simulink model "mc_power_model"  (R2022b)
settings: Solver=VariableStepAuto  StartTime=0.0  StopTime=5  FixedStep=1e-8  MaxStep=1e-7  RelTol=1e-3
undefined symbols (not defined in the file): f_s, find_system, Jm, Ki_ibat, Ki_id, Ki_iq, Kp_ibat, Kp_id, Kp_iq, Ld, limit_duty, Lq, p, Phi, Rs, Shunt, Snubber, Ts, U_dc, Vs_max
libraries: spsSeriesRLCBranchLib x12, spsCurrentMeasurementLib x9, spsVoltageMeasurementLib x7, spsMosfetLib x6, simulink x3, spsTriangleGeneratorLib x2, spsMeanLib x2, spsGroundLib x1, spsPermanentMagnetSynchronousMachineLib x1, spsDCVoltageSourceLib x1, spsThreePhaseVIMeasurementLib x1, spspowerguiLib x1
settings Model: Creator=ngoqu  LastModifiedBy=DoCongHieu
settings SolverCC: AlgebraicLoopSolver=TrustRegion
settings DataIOCC: ReturnWorkspaceOutputs=off
settings DebuggingCC: UnconnectedInputMsg=warning  UnconnectedOutputMsg=warning  UnconnectedLineMsg=warning  SFMachineParentedDataDiag=warning  ArithmeticOperatorsInVariantConditions=warning
settings ModelReferenceCC: EnableRefExpFcnMdlSchedulingChecks=on
settings SFSimCC: SimUseLocalCustomCode=off  CustomCodeUndefinedFunction=UseInterfaceOnly
settings RTWCC: RTWUseLocalCustomCode=off  DLArmComputeVersion=19.05

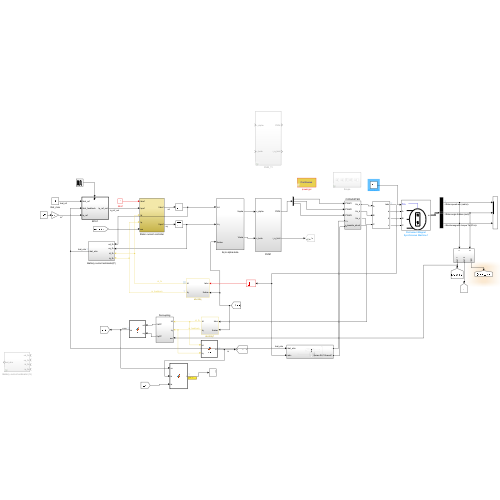
[thumbnail: Simulink's stored preview of the top-level diagram]
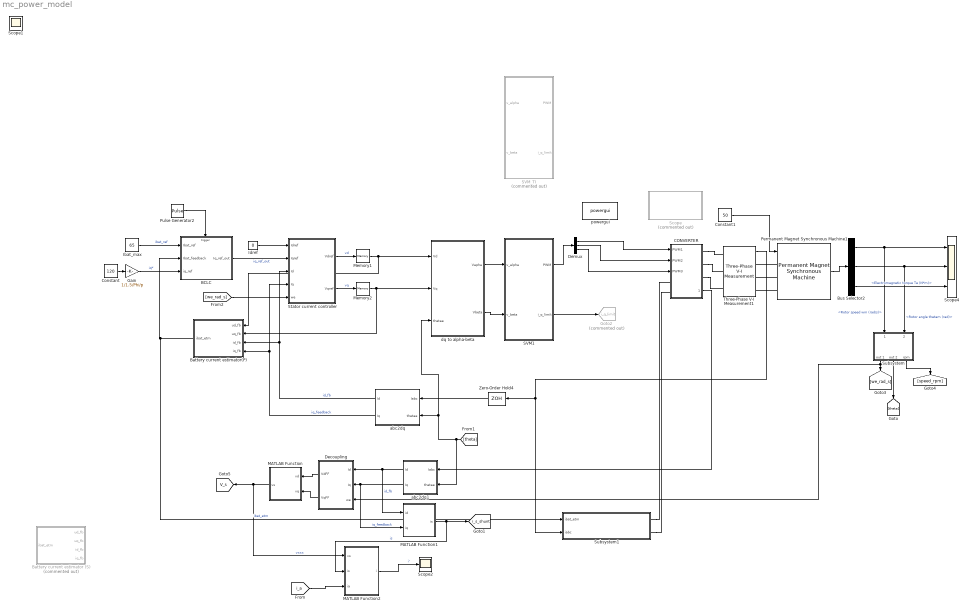
== system mc_power_model ==
  BCLC : Subsystem
  Battery current estimator (S) : Subsystem  Commented=on
  Battery current estimator(P) : Subsystem
  Bus Selector2 : BusSelector  OutputSignals=Rotor speed wm (rad/s),Rotor angle thetam (rad),Electromagnetic torque Te (N*m)
  CONVERTER : Subsystem  LoadFcn=find_system(gcs,'FollowLinks', 'on', 'LookUnderMasks', 'all');
      settings: PortSchema="{\"entries\":[{\"content\":{\"sides\":[{\"content\":{\"connectorIds\":[\"In1\",\"In2\",\"In3\",\"LConn1\",\"LConn2\"]},\"type\":\"ConnectorPlacement.EquallySpacedRectSide\",\"uuid\":\"f825b6ee-5639-4f6b-a9e2-a492c80e3f4f\"},{\"content\":{\"connectorIds\":[\"RConn1\",\"RConn2\",\"RConn3\",\"Out1\"],\"side\":\"RIGHT\"},\"type\":\"ConnectorPlacement.EquallySpacedRectSide\",\"uuid\":\"8c02666c-1fb3-4f32-9cc7-bf63baff1a79\"},{\"content\":{\"connectorIds\":[],\"side\":\"TOP\"},\"type\":\"ConnectorPlacement.EquallySpacedRectSide\",\"uuid\":\"503c9af4-c69d-4683-87ed-c435efd59e1b\"}]},\"type\":\"ConnectorPlacement.EquallySpacedConnector\",\"uuid\":\"38d4df0d-4e18-4d3b-af9f-c452f4b7a914\"}],\"packageUris\":[\"http://schema.mathworks.com/mf0/Connector/R2020b\"],\"version\":\"1.0\"}"
  Constant : Constant  Value=120
  Constant1 : Constant  Value=50
  Decoupling : Subsystem
  Demux : Demux  Outputs=3
  Gain : Gain  Gain=1/1.5/Phi/p
  Goto2 : Goto  Commented=on  GotoTag=i_q_limit  TagVisibility=global
  Ibat_max : Constant  Value=65
  Idref : Constant  Value=0  SampleTime=-1
  MATLAB Function : MATLAB Function  TreatAsAtomicUnit=on
  MATLAB Function1 : MATLAB Function  TreatAsAtomicUnit=on
  MATLAB Function2 : MATLAB Function  TreatAsAtomicUnit=on
  Memory1 : Memory  InheritSampleTime=on
  Memory2 : Memory  InheritSampleTime=on
  Permanent Magnet Synchronous Machine1 : spsPermanentMagnetSynchronousMachineLib/Permanent Magnet Synchronous Machine  NbPhases=3  FluxDistribution=Sinusoidal  RotorType=Salient-pole  MechanicalLoad=Torque Tm  PresetModel=No  ShowDetailedParameters=on  MeasurementBus=off  Resistance=Rs  Inductance=8.5e-3  dqInductances=[Ld Lq]  La=0.000395  MachineConstant=Flux linkage established by magnets (V.s)  Flux=Phi  VoltageCst=78.3561  TorqueCst=0.648  Flat=120  Mechanical=[Jm 0.000303448 p 0]  PolePairs=4  InitialConditions=[0,0, 0,0]  InitialConditions5ph=[0 0 0 0 0 0]  RefAngle=Aligned with phase A axis (original Park)  IterativeDiscreteModel=Trapezoidal non iterative  TsBlock=-1  TsPowergui=0
  Pulse Generator2 : DiscretePulseGenerator  PulseType=Time based  Period=1/1000  PulseWidth=50
  SVM1 : Subsystem
  SVM_TI : Subsystem  Commented=on
  Scope : Subsystem  Commented=on
  Scope2 : Scope
  Scope4 : Scope  NumInputPorts=3
  Stator current controller : Subsystem
  Subsystem : Subsystem
  Subsystem1 : Subsystem
  Three-Phase V-I Measurement1 : spsThreePhaseVIMeasurementLib/Three-Phase V-I Measurement  VoltageMeasurement=no  SetLabelV=off  LabelV=Vabc  Vpu=off  VpuLL=off  CurrentMeasurement=yes  SetLabelI=off  LabelI=Iabc  Ipu=off  Pbase=100e6  Vbase=500e3  OutputType=Complex  PhasorSimulation=off  PSBequivalent=0
  Zero-Order Hold4 : ZeroOrderHold  SampleTime=1/20000
  abc2dq : Subsystem
  abc2dq1 : Subsystem
  dq to alpha-beta : Subsystem
  powergui : spspowerguiLib/powergui  Priority=1  SimulationMode=Continuous  SampleTime=1/20000  frequency=60  Iterations=50  frequencyindice=0  Pbase=100e6  ErrMax=1e-4  UnitsV=kV  UnitsW=MW  buscounter=0  FunctionMessages=off  echomessages=off  EnableUseOfTLC=off  CurrentSourceSwitches=off  DisableSnubberDevices=off  DisableRonSwitches=off  DisableVfSwitches=off  DisplayEquations=off  AutomaticDiscreteSolvers=off  SolverType=Tustin/Backward Euler (TBE)  Interpol=off  ExternalGateDelay=off  methode=off  Ts=100  x0status=blocks  SPID=on  SwTol=0  HookPort=off  NonlinearTolerance=1e-4  nMaxIteration=100  ContinueOnMaxIteration=off  RestoreLinks=warning  ResistiveCurrentMeasurement=off  Frange=[0:2:500]  Ylog=off  Xlog=on  ShowGrid=off  save=off  variable=ZData  structure=0  ZoomFFT=off  StartTime=0.0  cycles=1  DisplayStyle=1  fundamental=60  FreqAxis=off  MaxFrequency=1000  frequencyindicesteady=1  RmsSteady=1  display=off
  Scope1 : Scope
  tag scope: V_s=global, i_s_shunt=global
  wires:
  abc2dq/1(Id) -> Stator current controller/3(Id), Battery current estimator(P)/3(id_fb)  "id_fb"
  Idref/1 -> Stator current controller/1(Idref)
  [theta] -> abc2dq1/2(thetae), dq to alpha-beta/3(thetae), abc2dq/2(thetae)
  Stator current controller/2(Vqref) -> Memory2/1  "vq"
  Stator current controller/1(Vdref) -> Memory1/1  "vd"
  SVM1/1(PWM) -> Demux/1
  dq to alpha-beta/2(Vbeta) -> SVM1/2(v_beta)
  dq to alpha-beta/1(Vapha) -> SVM1/1(v_alpha)
  Zero-Order Hold4/1 -> abc2dq/1(Iabc)
  Memory1/1 -> dq to alpha-beta/1(Vd), Battery current estimator(P)/1(ud_fb)
  SVM1/2(i_q_limit) -> Goto2/1
  Subsystem/3(rpm) -> [speed_rpm]
  Bus Selector2/1 -> Subsystem/1("1 "), Scope4/1  "<Rotor speed wm (rad/s)>"
  Subsystem/1(out 1) -> Decoupling/3(we), [we_rad_s]
  Subsystem/2("out 2 ") -> [theta]
  Permanent Magnet Synchronous Machine1/1 -> Bus Selector2/1
  Bus Selector2/2 -> Subsystem/2(2), Scope4/2  "<Rotor angle thetam (rad)>"
  Bus Selector2/3 -> Scope4/3  "<Electromagnetic torque Te (N*m)>"
  [we_rad_s] -> Stator current controller/5(we)
  abc2dq/2(Iq) -> Stator current controller/4(Iq), Battery current estimator(P)/4(iq_fb)  "iq_feedback"
  Ibat_max/1 -> BCLC/1(Ibat_ref)  "ibat_ref"
  Gain/1 -> BCLC/3(iq_ref)  "iq*"
  Pulse Generator2/1 -> BCLC/Trigger
  Battery current estimator(P)/1(ibat_etm) -> Subsystem1/1(ibat_etm), BCLC/2(Ibat_feedback)  "ibat_etm"
  Demux/1 -> CONVERTER/1(PWM1)
  Demux/2 -> CONVERTER/2(PWM2)
  Demux/3 -> CONVERTER/3(PWM3)
  Memory2/1 -> dq to alpha-beta/2(Vq), Battery current estimator(P)/2(uq_fb)
  Constant/1 -> Gain/1
  BCLC/1(Iq_ref_out) -> Stator current controller/2(Iqref)  "iq_ref_out"
  Constant1/1 -> Permanent Magnet Synchronous Machine1/1
  MATLAB Function/1(vs) -> MATLAB Function2/1(vs), [V_s]  "vxxx"
  MATLAB Function1/1(is) -> MATLAB Function2/2(is), [i_s_shunt]  "is"
  Three-Phase V-I Measurement1/1 -> Subsystem1/2(iabc), Zero-Order Hold4/1
  CONVERTER/1(Iabc_lowside_shunt) -> abc2dq1/1(Iabc)
  abc2dq1/1(Id) -> Decoupling/1(Id), MATLAB Function1/1(id)  "id_fb"
  abc2dq1/2(Iq) -> Decoupling/2(Iq), MATLAB Function1/2(iq)  "iq_feedback"
  Decoupling/1(VdFF) -> MATLAB Function/1(vd)
  Decoupling/2(VqFF) -> MATLAB Function/2(vq)
  [i_a] -> MATLAB Function2/3(ia)
  MATLAB Function2/1(i) -> Scope2/1  "i'"
  connections:
  CONVERTER/RConn3 -- Three-Phase V-I Measurement1/LConn3
  Permanent Magnet Synchronous Machine1/LConn3 -- Three-Phase V-I Measurement1/RConn3
  Permanent Magnet Synchronous Machine1/LConn2 -- Three-Phase V-I Measurement1/RConn2
  Permanent Magnet Synchronous Machine1/LConn1 -- Three-Phase V-I Measurement1/RConn1
  CONVERTER/RConn1 -- Three-Phase V-I Measurement1/LConn1
  CONVERTER/RConn2 -- Three-Phase V-I Measurement1/LConn2
  Subsystem1/RConn1 -- CONVERTER/LConn1
  Subsystem1/RConn2 -- CONVERTER/LConn2

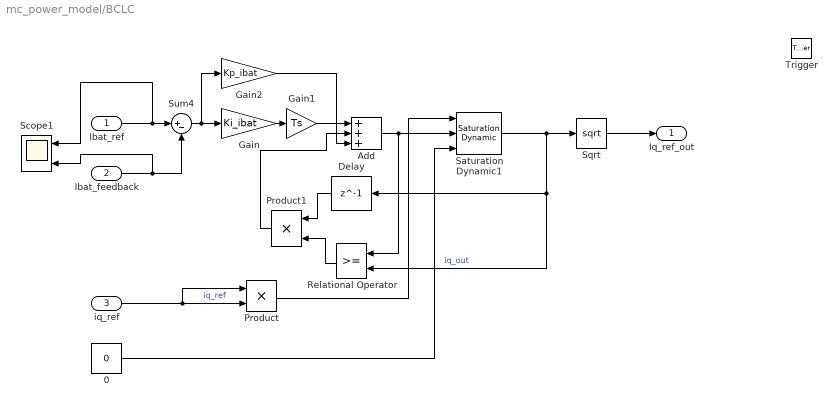
== system mc_power_model/BCLC ==
  Ibat_ref : Inport
  Ibat_feedback : Inport  Port=2
  iq_ref : Inport  Port=3
  Trigger : TriggerPort  VariantControl=Variant
  0 : Constant  Value=0
  Add : Sum  Inputs=+++
  Delay : Delay  DelayLength=1
  Gain : Gain  Gain=Ki_ibat
  Gain1 : Gain  Gain=Ts
  Gain2 : Gain  Gain=Kp_ibat
  Product : Product
  Product1 : Product
  Relational Operator : RelationalOperator  OutDataTypeStr=boolean  RndMeth=Simplest  InputSameDT=off
  Saturation Dynamic1 : simulink/Discontinuities/Saturation Dynamic  OutMin=[]  OutMax=[]  OutDataTypeStr=Inherit: Same as second input  OutDataType=fixdt(1, 16)  OutScaling=2^-10  DoSatur=off
  Scope1 : Scope  NumInputPorts=2
  Sqrt : Sqrt
  Sum4 : Sum  Inputs=|+-
  Iq_ref_out : Outport  VectorParamsAs1DForOutWhenUnconnected=off
  wires:
  Sqrt/1 -> Iq_ref_out/1
  0/1 -> Saturation Dynamic1/3
  Saturation Dynamic1/1 -> Relational Operator/2, Delay/1, Sqrt/1  "iq_out"
  Sum4/1 -> Gain2/1, Gain/1
  Ibat_feedback/1 -> Scope1/2, Sum4/2
  Gain/1 -> Gain1/1
  Add/1 -> Relational Operator/1, Saturation Dynamic1/2
  Gain1/1 -> Add/1
  iq_ref/1 -> Product/2, Product/1  "iq_ref"
  Product/1 -> Saturation Dynamic1/1
  Gain2/1 -> Add/3
  Delay/1 -> Product1/1
  Product1/1 -> Add/2
  Relational Operator/1 -> Product1/2
  Ibat_ref/1 -> Scope1/1, Sum4/1

== system mc_power_model/Battery current estimator (S) ==
  ud_fb : Inport
  uq_fb : Inport  Port=2
  id_fb : Inport  Port=3
  iq_fb : Inport  Port=4
  Constant : Constant  Value=U_dc
  Estimate ibattery : MATLAB Function  TreatAsAtomicUnit=on
  Zero-Order Hold2 : ZeroOrderHold  SampleTime=1/1000
  ibat_etm : Outport  VectorParamsAs1DForOutWhenUnconnected=off
  wires:
  Constant/1 -> Estimate ibattery/5(udc)
  id_fb/1 -> Estimate ibattery/1(id_fb)
  uq_fb/1 -> Estimate ibattery/4(uq_sp)
  Estimate ibattery/1(ibat_etm) -> Zero-Order Hold2/1
  ud_fb/1 -> Estimate ibattery/3(ud_sp)
  iq_fb/1 -> Estimate ibattery/2(iq_fb)
  Zero-Order Hold2/1 -> ibat_etm/1

== system mc_power_model/Battery current estimator(P) ==
  ud_fb : Inport
  uq_fb : Inport  Port=2
  id_fb : Inport  Port=3
  iq_fb : Inport  Port=4
  Constant : Constant  Value=U_dc
  Estimate ibattery : MATLAB Function  TreatAsAtomicUnit=on
  Zero-Order Hold2 : ZeroOrderHold  SampleTime=1/1000
  ibat_etm : Outport  VectorParamsAs1DForOutWhenUnconnected=off
  wires:
  Constant/1 -> Estimate ibattery/5(udc)
  id_fb/1 -> Estimate ibattery/1(id_fb)
  uq_fb/1 -> Estimate ibattery/4(uq_sp)
  Estimate ibattery/1(ibat_etm) -> Zero-Order Hold2/1
  ud_fb/1 -> Estimate ibattery/3(ud_sp)
  iq_fb/1 -> Estimate ibattery/2(iq_fb)
  Zero-Order Hold2/1 -> ibat_etm/1

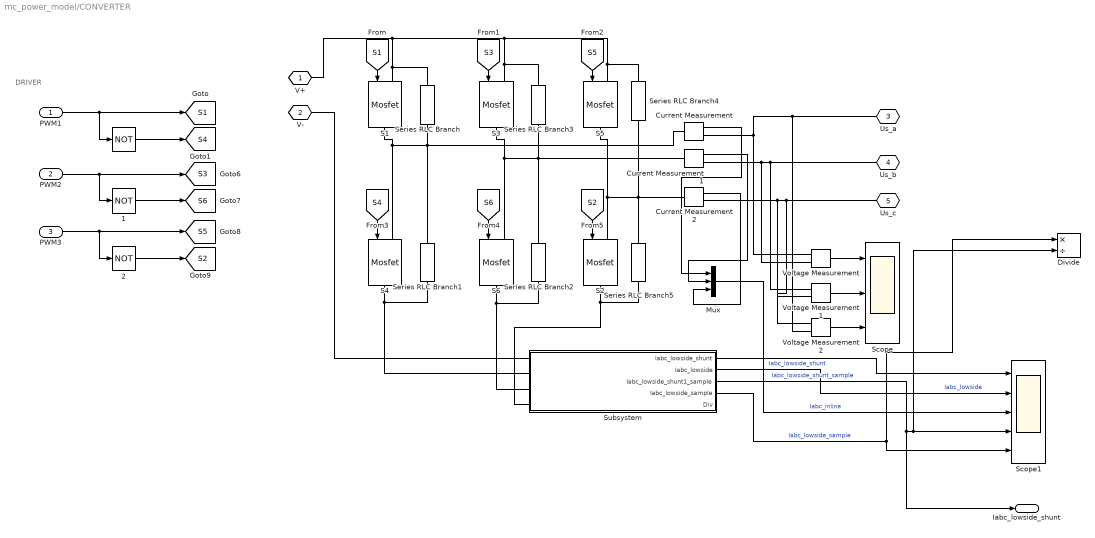
== system mc_power_model/CONVERTER ==
  note: DRIVER
  PWM1 : Inport
  PWM2 : Inport  Port=2
  PWM3 : Inport  Port=3
  "     " : Logic  Operator=NOT  AllPortsSameDT=off  OutDataTypeStr=boolean
  "     1" : Logic  Operator=NOT  AllPortsSameDT=off  OutDataTypeStr=boolean
  "     2" : Logic  Operator=NOT  AllPortsSameDT=off  OutDataTypeStr=boolean
  Current Measurement : spsCurrentMeasurementLib/Current Measurement  PhasorSimulation=off  OutputType=Complex  PSBequivalent=0
  Current Measurement1 : spsCurrentMeasurementLib/Current Measurement  PhasorSimulation=off  OutputType=Complex  PSBequivalent=0
  Current Measurement2 : spsCurrentMeasurementLib/Current Measurement  PhasorSimulation=off  OutputType=Complex  PSBequivalent=0
  Divide : Product  Inputs=*/
  Mux : Mux  Inputs=3
  S{1..6} (6 alike) : spsMosfetLib/Mosfet  Ron=0.001  Lon=0  Rd=0.01  Vfd=1.3  IC=0  Rs=1e5  Cs=inf  Measurements=off
  Scope : Scope  NumInputPorts=3
  Scope1 : Scope  NumInputPorts=5
  Series RLC Branch{,1..5} (6 alike) : spsSeriesRLCBranchLib/Series RLC Branch  LConnTagsString=__new0  RConnTagsString=__new0  BranchType=RC  Resistance=Snubber.R  Inductance=1e-3  SetiL0=off  InitialCurrent=0  Capacitance=Snubber.C  Setx0=off  InitialVoltage=0  Measurements=None
  Subsystem : Subsystem
  Voltage Measurement : spsVoltageMeasurementLib/Voltage Measurement  PhasorSimulation=off  OutputType=Complex  PSBequivalent=0
  Voltage Measurement1 : spsVoltageMeasurementLib/Voltage Measurement  PhasorSimulation=off  OutputType=Complex  PSBequivalent=0
  Voltage Measurement2 : spsVoltageMeasurementLib/Voltage Measurement  PhasorSimulation=off  OutputType=Complex  PSBequivalent=0
  V+ : PMIOPort  Tag=PMCPort  Side=Left
  V- : PMIOPort  Tag=PMCPort  Port=2  Side=Left
  Us_a : PMIOPort  Tag=PMCPort  Port=3  Side=Right
  Us_b : PMIOPort  Tag=PMCPort  Port=4  Side=Right
  Us_c : PMIOPort  Tag=PMCPort  Port=5  Side=Right
  Iabc_lowside_shunt : Outport
  tag scope: S1=global, S2=global, S3=global, S4=global, S5=global, S6=global
  wires:
  Voltage Measurement/1 -> Scope/1
  [S3] -> S3/1
  [S4] -> S4/1
  [S2] -> S2/1
  [S1] -> S1/1
  [S5] -> S5/1
  [S6] -> S6/1
  PWM1/1 -> "     "/1, [S1]
  "     "/1 -> [S4]
  "     1"/1 -> [S6]
  PWM2/1 -> [S3], "     1"/1
  PWM3/1 -> "     2"/1, [S5]
  "     2"/1 -> [S2]
  Voltage Measurement1/1 -> Scope/2
  Voltage Measurement2/1 -> Scope/3
  Subsystem/1(Iabc_lowside_shunt) -> Scope1/1  "Iabc_lowside_shunt"
  Subsystem/2(Iabc_lowside) -> Scope1/2  "Iabc_lowside"
  Current Measurement1/1 -> Mux/2
  Current Measurement/1 -> Mux/1
  Current Measurement2/1 -> Mux/3
  Mux/1 -> Scope1/3  "Iabc_inline"
  Subsystem/3(Iabc_lowside_shunt1_sample) -> Divide/2, Scope1/4, Iabc_lowside_shunt/1  "Iabc_lowside_shunt_sample"
  Subsystem/4(Iabc_lowside_sample) -> Scope1/5, Divide/1  "Iabc_lowside_sample"
  connections:
  Voltage Measurement2/LConn1 -- Current Measurement2/RConn1 -- Voltage Measurement1/LConn2 -- Us_c/RConn1
  S5/LConn1 -- Series RLC Branch4/LConn1 -- Series RLC Branch/LConn1 -- S1/LConn1 -- V+/RConn1 -- Series RLC Branch3/LConn1 -- S3/LConn1
  Voltage Measurement2/LConn2 -- Us_a/RConn1 -- Current Measurement/RConn1 -- Voltage Measurement/LConn1
  Voltage Measurement/LConn2 -- Voltage Measurement1/LConn1 -- Us_b/RConn1 -- Current Measurement1/RConn1
  V-/RConn1 -- Subsystem/LConn1
  S4/RConn1 -- Series RLC Branch1/RConn1 -- Subsystem/LConn2
  Subsystem/LConn3 -- Series RLC Branch2/RConn1 -- S6/RConn1
  S2/RConn1 -- Series RLC Branch5/RConn1 -- Subsystem/LConn4
  S4/LConn1 -- S1/RConn1 -- Series RLC Branch/RConn1 -- Current Measurement/LConn1 -- Series RLC Branch1/LConn1
  S6/LConn1 -- Series RLC Branch3/RConn1 -- Series RLC Branch2/LConn1 -- Current Measurement1/LConn1 -- S3/RConn1
  S2/LConn1 -- Series RLC Branch4/RConn1 -- Current Measurement2/LConn1 -- Series RLC Branch5/LConn1 -- S5/RConn1

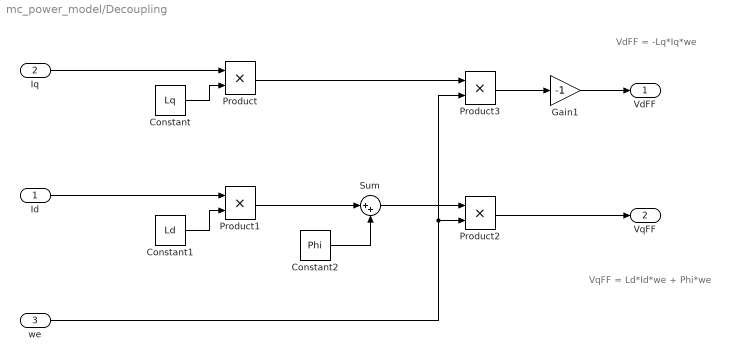
== system mc_power_model/Decoupling ==
  note: VqFF = Ld*Id*we + Phi*we
  note: VdFF = -Lq*Iq*we
  Id : Inport
  Iq : Inport  Port=2
  we : Inport  Port=3
  Constant : Constant  Value=Lq
  Constant1 : Constant  Value=Ld
  Constant2 : Constant  Value=Phi
  Gain1 : Gain  Gain=-1
  Product{,1..3} (4 alike) : Product
  Sum : Sum  Inputs=|++
  VdFF : Outport  VectorParamsAs1DForOutWhenUnconnected=off
  VqFF : Outport  Port=2  VectorParamsAs1DForOutWhenUnconnected=off
  wires:
  Product2/1 -> VqFF/1
  Gain1/1 -> VdFF/1
  Product/1 -> Product3/1
  Product3/1 -> Gain1/1
  Constant/1 -> Product/2
  Iq/1 -> Product/1
  Id/1 -> Product1/1
  Constant1/1 -> Product1/2
  Sum/1 -> Product2/1
  Constant2/1 -> Sum/2
  Product1/1 -> Sum/1
  we/1 -> Product2/2, Product3/2

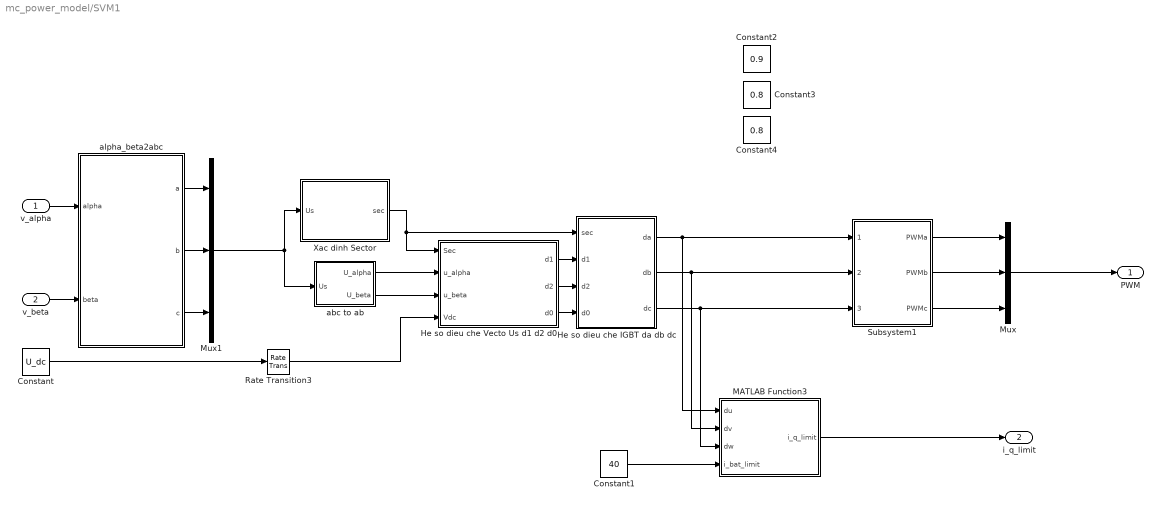
== system mc_power_model/SVM1 ==
  v_alpha : Inport
  v_beta : Inport  Port=2
  Constant : Constant  Value=U_dc
  Constant1 : Constant  Value=40
  Constant2 : Constant  Value=0.9
  Constant3 : Constant  Value=0.8
  Constant4 : Constant  Value=0.8
  He so dieu che IGBT da db dc : MATLAB Function  TreatAsAtomicUnit=on
  He so dieu che Vecto Us d1 d2 d0 : MATLAB Function  TreatAsAtomicUnit=on
  MATLAB Function3 : MATLAB Function  TreatAsAtomicUnit=on
  Mux : Mux  Inputs=3
  Mux1 : Mux  Inputs=3
  Rate Transition3 : RateTransition
  Subsystem1 : Subsystem
  Xac dinh Sector : MATLAB Function  TreatAsAtomicUnit=on
  abc to ab : Subsystem
  alpha_beta2abc : Subsystem
  PWM : Outport  VectorParamsAs1DForOutWhenUnconnected=off
  i_q_limit : Outport  Port=2  VectorParamsAs1DForOutWhenUnconnected=off
  wires:
  alpha_beta2abc/3(c) -> Mux1/3
  alpha_beta2abc/2(b) -> Mux1/2
  alpha_beta2abc/1(a) -> Mux1/1
  v_alpha/1 -> alpha_beta2abc/1(alpha)
  v_beta/1 -> alpha_beta2abc/2(beta)
  Mux1/1 -> Xac dinh Sector/1(Us), abc to ab/1(Us)
  He so dieu che Vecto Us d1 d2 d0/2(d2) -> He so dieu che IGBT da db dc/3(d2)
  He so dieu che Vecto Us d1 d2 d0/3(d0) -> He so dieu che IGBT da db dc/4(d0)
  He so dieu che Vecto Us d1 d2 d0/1(d1) -> He so dieu che IGBT da db dc/2(d1)
  Xac dinh Sector/1(sec) -> He so dieu che Vecto Us d1 d2 d0/1(Sec), He so dieu che IGBT da db dc/1(sec)
  abc to ab/2(U_beta) -> He so dieu che Vecto Us d1 d2 d0/3(u_beta)
  abc to ab/1(U_alpha) -> He so dieu che Vecto Us d1 d2 d0/2(u_alpha)
  Constant/1 -> Rate Transition3/1
  Mux/1 -> PWM/1
  Rate Transition3/1 -> He so dieu che Vecto Us d1 d2 d0/4(Vdc)
  He so dieu che IGBT da db dc/1(da) -> Subsystem1/1(1), MATLAB Function3/1(du)
  He so dieu che IGBT da db dc/2(db) -> Subsystem1/2(2), MATLAB Function3/2(dv)
  He so dieu che IGBT da db dc/3(dc) -> Subsystem1/3(3), MATLAB Function3/3(dw)
  Subsystem1/1(PWMa) -> Mux/1
  Subsystem1/2(PWMb) -> Mux/2
  Subsystem1/3(PWMc) -> Mux/3
  Constant1/1 -> MATLAB Function3/4(i_bat_limit)
  MATLAB Function3/1(i_q_limit) -> i_q_limit/1

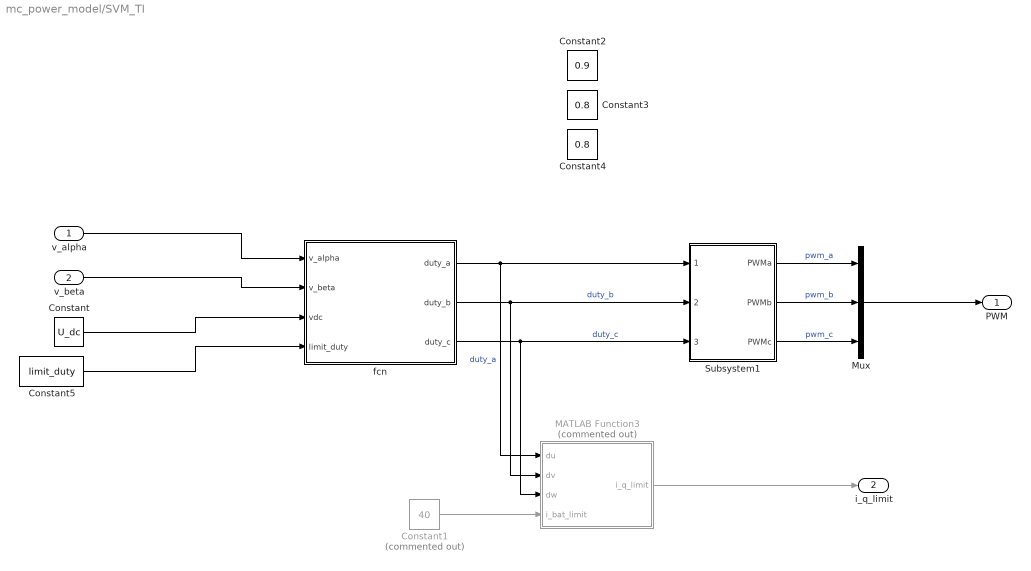
== system mc_power_model/SVM_TI ==
  v_alpha : Inport
  v_beta : Inport  Port=2
  Constant : Constant  Value=U_dc
  Constant1 : Constant  Commented=on  Value=40
  Constant2 : Constant  Value=0.9
  Constant3 : Constant  Value=0.8
  Constant4 : Constant  Value=0.8
  Constant5 : Constant  Value=limit_duty
  MATLAB Function3 : MATLAB Function  Commented=on  TreatAsAtomicUnit=on
  Mux : Mux  Inputs=3
  Subsystem1 : Subsystem
  fcn : MATLAB Function  TreatAsAtomicUnit=on
  PWM : Outport  VectorParamsAs1DForOutWhenUnconnected=off
  i_q_limit : Outport  Port=2  VectorParamsAs1DForOutWhenUnconnected=off
  wires:
  v_alpha/1 -> fcn/1(v_alpha)
  v_beta/1 -> fcn/2(v_beta)
  Mux/1 -> PWM/1
  fcn/1(duty_a) -> Subsystem1/1(1), MATLAB Function3/1(du)  "duty_a"
  fcn/2(duty_b) -> Subsystem1/2(2), MATLAB Function3/2(dv)  "duty_b"
  fcn/3(duty_c) -> Subsystem1/3(3), MATLAB Function3/3(dw)  "duty_c"
  Subsystem1/1(PWMa) -> Mux/1  "pwm_a"
  Subsystem1/2(PWMb) -> Mux/2  "pwm_b"
  Subsystem1/3(PWMc) -> Mux/3  "pwm_c"
  Constant1/1 -> MATLAB Function3/4(i_bat_limit)
  MATLAB Function3/1(i_q_limit) -> i_q_limit/1
  Constant/1 -> fcn/3(vdc)
  Constant5/1 -> fcn/4(limit_duty)

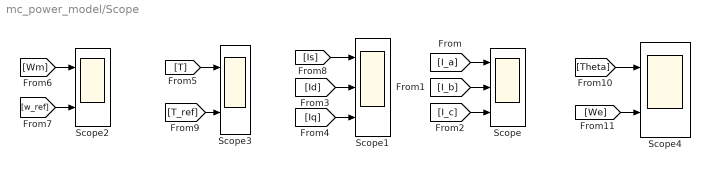
== system mc_power_model/Scope ==
  Scope : Scope  NumInputPorts=3
  Scope1 : Scope  NumInputPorts=3
  Scope2 : Scope  NumInputPorts=2
  Scope3 : Scope  NumInputPorts=2
  Scope4 : Scope  NumInputPorts=2
  wires:
  [I_a] -> Scope/1
  [I_c] -> Scope/3
  [I_b] -> Scope/2
  [Wm] -> Scope2/1
  [w_ref] -> Scope2/2
  [T] -> Scope3/1
  [T_ref] -> Scope3/2
  [Theta] -> Scope4/1
  [We] -> Scope4/2
  [Id] -> Scope1/2
  [Iq] -> Scope1/3
  [Is] -> Scope1/1

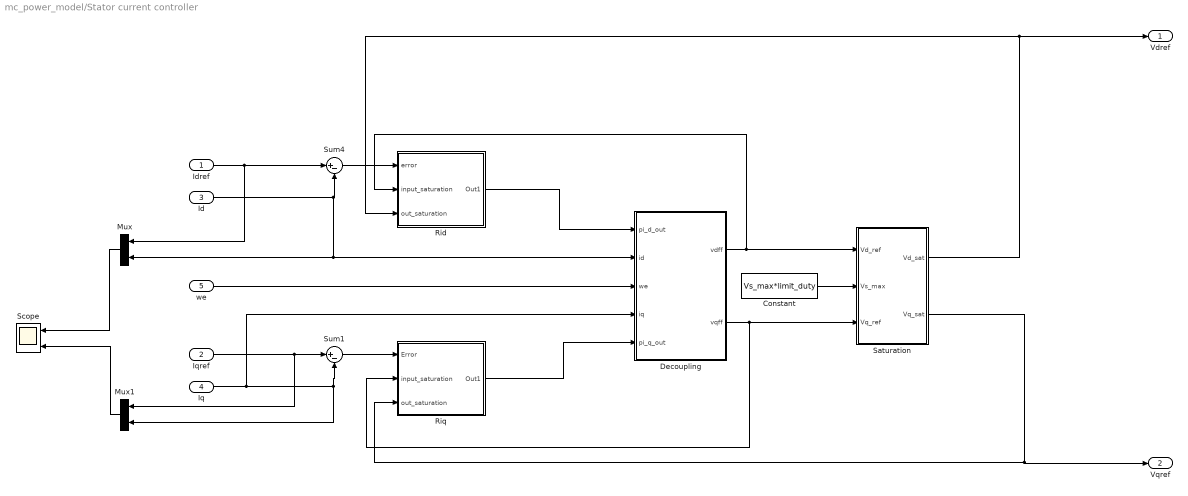
== system mc_power_model/Stator current controller ==
  Idref : Inport
  Iqref : Inport  Port=2
  Id : Inport  Port=3
  Iq : Inport  Port=4
  we : Inport  Port=5
  Constant : Constant  Value=Vs_max*limit_duty
  Decoupling : Subsystem
  Mux : Mux  Inputs=2
  Mux1 : Mux  Inputs=2
  Rid : Subsystem
  Riq : Subsystem
  Saturation : Subsystem
  Scope : Scope  NumInputPorts=2
  Sum1 : Sum  Inputs=|+-
  Sum4 : Sum  Inputs=|+-
  Vdref : Outport  VectorParamsAs1DForOutWhenUnconnected=off
  Vqref : Outport  Port=2  VectorParamsAs1DForOutWhenUnconnected=off
  wires:
  Constant/1 -> Saturation/2(Vs_max)
  Mux1/1 -> Scope/2
  Mux/1 -> Scope/1
  Id/1 -> Decoupling/2(id), Mux/2, Sum4/2
  Iq/1 -> Decoupling/4(iq), Sum1/2, Mux1/2
  Iqref/1 -> Mux1/1, Sum1/1
  Idref/1 -> Sum4/1, Mux/1
  Decoupling/2(vqff) -> Riq/2(input_saturation), Saturation/3(Vq_ref)
  Decoupling/1(vdff) -> Rid/2(input_saturation), Saturation/1(Vd_ref)
  we/1 -> Decoupling/3(we)
  Sum4/1 -> Rid/1(error)
  Rid/1(Out1) -> Decoupling/1(pi_d_out)
  Sum1/1 -> Riq/1(Error)
  Riq/1(Out1) -> Decoupling/5(pi_q_out)
  Saturation/1(Vd_sat) -> Vdref/1, Rid/3(out_saturation)
  Saturation/2(Vq_sat) -> Vqref/1, Riq/3(out_saturation)

== system mc_power_model/Subsystem ==
  "1 " : Inport
  2 : Inport  Port=2
  Constant : Constant  Value=-10/180*3.14
  Constant1 : Constant  Value=0
  PolePairs : Gain  Gain=p
  PolePairs1 : Gain  Gain=p
  PolePairs2 : Gain  Gain=9.55
  Subtract : Sum  Inputs=+-
  out 1 : Outport  VectorParamsAs1DForOutWhenUnconnected=off
  "out 2 " : Outport  Port=2  VectorParamsAs1DForOutWhenUnconnected=off
  rpm : Outport  Port=3  VectorParamsAs1DForOutWhenUnconnected=off
  wires:
  "1 "/1 -> PolePairs2/1, PolePairs1/1
  2/1 -> PolePairs/1
  PolePairs1/1 -> out 1/1
  PolePairs2/1 -> rpm/1
  PolePairs/1 -> Subtract/1
  Subtract/1 -> "out 2 "/1
  Constant1/1 -> Subtract/2

== system mc_power_model/Subsystem1 ==
  ibat_etm : Inport
  iabc : Inport  Port=2
  Abs2 : Abs  SaturateOnIntegerOverflow=off
  Current Measurement2 : spsCurrentMeasurementLib/Current Measurement  PhasorSimulation=off  OutputType=Complex  PSBequivalent=0
  Current Measurement3 : spsCurrentMeasurementLib/Current Measurement  PhasorSimulation=off  OutputType=Complex  PSBequivalent=0
  Mean : spsMeanLib/Mean  Freq=50  Vinit=0  Ts=1/100000
  Mean1 : spsMeanLib/Mean  Freq=50  Vinit=0  Ts=1/100000
  Mux : Mux  Inputs=7
  Scope6 : Scope
  Series RLC Branch2 : spsSeriesRLCBranchLib/Series RLC Branch  LConnTagsString=__new0  RConnTagsString=__new0  BranchType=RC  Resistance=0.026/4  Inductance=1e-3  SetiL0=off  InitialCurrent=0  Capacitance=4*390e-6  Setx0=off  InitialVoltage=0  Measurements=None
  Series RLC Branch3 : spsSeriesRLCBranchLib/Series RLC Branch  LConnTagsString=__new0  RConnTagsString=__new0  BranchType=R  Resistance=0.04  Inductance=1e-3  SetiL0=off  InitialCurrent=0  Capacitance=1e-3  Setx0=off  InitialVoltage=0  Measurements=None
  Udc V1 : spsDCVoltageSourceLib/DC Voltage Source  Amplitude=U_dc  Measurements=Voltage
  - : PMIOPort  Side=Right
  Series RLC Branch1 : PMIOPort  Port=2  Side=Right
  wires:
  ibat_etm/1 -> Mux/6
  Mean1/1 -> Mux/2  "i_ivt_filter"
  Mean/1 -> Mux/4  "ibat_filter"
  Current Measurement3/1 -> Mean/1, Mux/3  "i_battery"
  Current Measurement2/1 -> Mean1/1, Mux/1  "i_inveter"
  Mux/1 -> Scope6/1
  Abs2/1 -> Mux/7
  iabc/1 -> Abs2/1
  connections:
  Series RLC Branch3/LConn1 -- Udc V1/LConn1
  Current Measurement3/RConn1 -- Series RLC Branch2/LConn1 -- Current Measurement2/LConn1
  Series RLC Branch2/RConn1 -- Series RLC Branch1/RConn1 -- Series RLC Branch3/RConn1
  Current Measurement3/LConn1 -- Udc V1/RConn1
  Current Measurement2/RConn1 -- -/RConn1

== system mc_power_model/abc2dq ==
  note: Iq
  note: Id
  note: Ib
  note: Ia
  note: Ibeta
  note: Ialpha
  Iabc : Inport
  thetae : Inport  Port=2
  Demux : Demux  Outputs=3
  Fcn : Fcn  Expr=1/sqrt(3)*(u(1)+2*u(2))
  Fcn1 : Fcn  Expr=u(1)*cos(u(3))+u(2)*sin(u(3))
  Fcn2 : Fcn  Expr=-u(1)*sin(u(3))+u(2)*cos(u(3))
  Mux : Mux  Inputs=2
  Mux1 : Mux  Inputs=3
  Mux2 : Mux  Inputs=3
  Terminator1 : Terminator
  Zero-Order Hold1 : ZeroOrderHold  SampleTime=1/20000
  Zero-Order Hold2 : ZeroOrderHold  SampleTime=1/20000
  Id : Outport  VectorParamsAs1DForOutWhenUnconnected=off
  Iq : Outport  Port=2  VectorParamsAs1DForOutWhenUnconnected=off
  wires:
  Iabc/1 -> Demux/1
  Demux/2 -> Mux/2
  Demux/3 -> Terminator1/1
  Mux/1 -> Fcn/1
  Mux1/1 -> Fcn1/1
  Mux2/1 -> Fcn2/1
  Demux/1 -> Mux2/1, Mux1/1, Mux/1
  Fcn/1 -> Mux2/2, Mux1/2
  thetae/1 -> Mux1/3, Mux2/3
  Fcn1/1 -> Zero-Order Hold2/1
  Fcn2/1 -> Zero-Order Hold1/1
  Zero-Order Hold2/1 -> Id/1
  Zero-Order Hold1/1 -> Iq/1

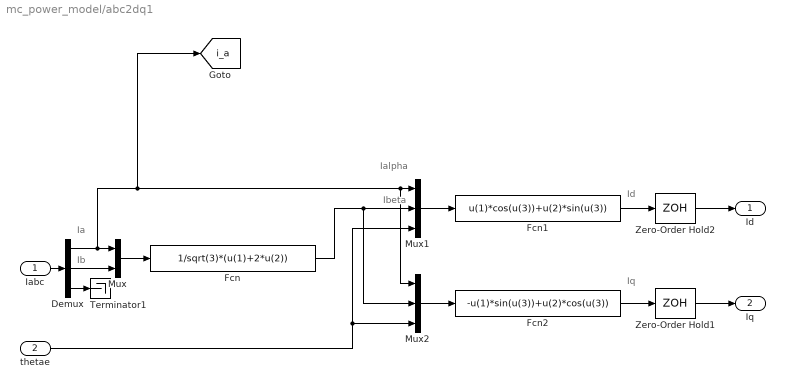
== system mc_power_model/abc2dq1 ==
  note: Iq
  note: Id
  note: Ib
  note: Ia
  note: Ibeta
  note: Ialpha
  Iabc : Inport
  thetae : Inport  Port=2
  Demux : Demux  Outputs=3
  Fcn : Fcn  Expr=1/sqrt(3)*(u(1)+2*u(2))
  Fcn1 : Fcn  Expr=u(1)*cos(u(3))+u(2)*sin(u(3))
  Fcn2 : Fcn  Expr=-u(1)*sin(u(3))+u(2)*cos(u(3))
  Mux : Mux  Inputs=2
  Mux1 : Mux  Inputs=3
  Mux2 : Mux  Inputs=3
  Terminator1 : Terminator
  Zero-Order Hold1 : ZeroOrderHold  SampleTime=1/20000
  Zero-Order Hold2 : ZeroOrderHold  SampleTime=1/20000
  Id : Outport  VectorParamsAs1DForOutWhenUnconnected=off
  Iq : Outport  Port=2  VectorParamsAs1DForOutWhenUnconnected=off
  tag scope: i_a=global
  wires:
  Iabc/1 -> Demux/1
  Demux/2 -> Mux/2
  Demux/3 -> Terminator1/1
  Mux/1 -> Fcn/1
  Mux1/1 -> Fcn1/1
  Mux2/1 -> Fcn2/1
  Demux/1 -> [i_a], Mux2/1, Mux1/1, Mux/1
  Fcn/1 -> Mux2/2, Mux1/2
  thetae/1 -> Mux1/3, Mux2/3
  Fcn1/1 -> Zero-Order Hold2/1
  Fcn2/1 -> Zero-Order Hold1/1
  Zero-Order Hold2/1 -> Id/1
  Zero-Order Hold1/1 -> Iq/1

== system mc_power_model/dq to alpha-beta ==
  note: Vbeta
  note: Valpha
  Vd : Inport
  Vq : Inport  Port=2
  thetae : Inport  Port=3
  Fcn : Fcn  Expr=u(1)*cos(u(3))-u(2)*sin(u(3))
  Fcn1 : Fcn  Expr=u(1)*sin(u(3))+u(2)*cos(u(3))
  Mux : Mux  Inputs=3
  Mux1 : Mux  Inputs=3
  Vapha : Outport  VectorParamsAs1DForOutWhenUnconnected=off
  Vbeta : Outport  Port=2  VectorParamsAs1DForOutWhenUnconnected=off
  wires:
  Vd/1 -> Mux1/1, Mux/1
  thetae/1 -> Mux1/3, Mux/3
  Mux/1 -> Fcn/1
  Mux1/1 -> Fcn1/1
  Vq/1 -> Mux1/2, Mux/2
  Fcn/1 -> Vapha/1
  Fcn1/1 -> Vbeta/1

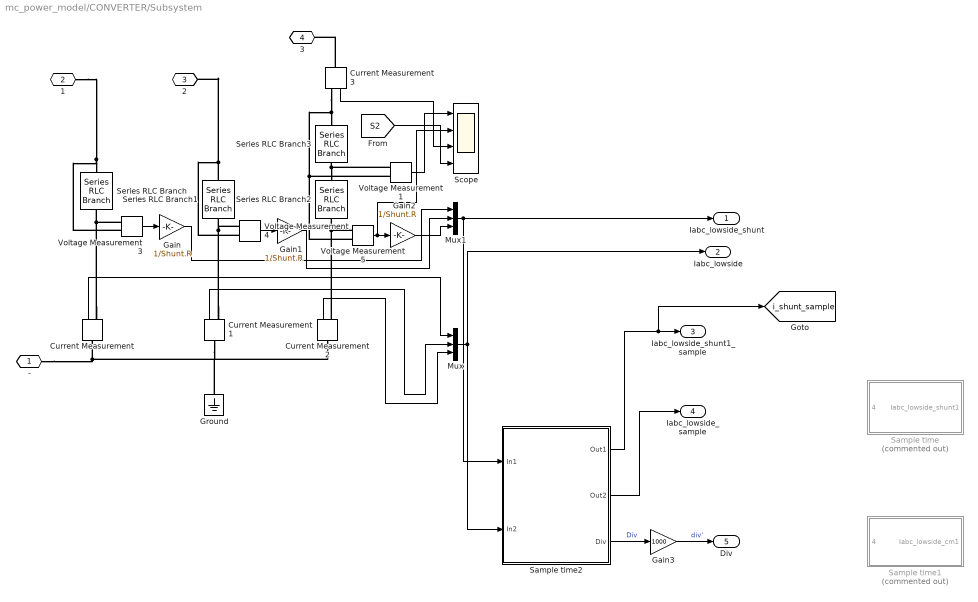
== system mc_power_model/CONVERTER/Subsystem ==
  Current Measurement{,1..3} (4 alike) : spsCurrentMeasurementLib/Current Measurement  PhasorSimulation=off  OutputType=Complex  PSBequivalent=0
  Gain : Gain  Gain=1/Shunt.R
  Gain1 : Gain  Gain=1/Shunt.R
  Gain2 : Gain  Gain=1/Shunt.R
  Gain3 : Gain  Gain=1000
  Ground : spsGroundLib/Ground  LConnTagsString=a
  Mux : Mux  Inputs=3
  Mux1 : Mux  Inputs=3
  Sample time : Subsystem  Commented=on
  Sample time1 : Subsystem  Commented=on
  Sample time2 : Subsystem
  Scope : Scope  NumInputPorts=4
  Series RLC Branch : spsSeriesRLCBranchLib/Series RLC Branch  LConnTagsString=__new0  RConnTagsString=__new0  BranchType=RL  Resistance=Shunt.R  Inductance=Shunt.L  SetiL0=off  InitialCurrent=0  Capacitance=1e-6  Setx0=off  InitialVoltage=0  Measurements=None
  Series RLC Branch1 : spsSeriesRLCBranchLib/Series RLC Branch  LConnTagsString=__new0  RConnTagsString=__new0  BranchType=RL  Resistance=Shunt.R  Inductance=Shunt.L  SetiL0=off  InitialCurrent=0  Capacitance=1e-6  Setx0=off  InitialVoltage=0  Measurements=None
  Series RLC Branch2 : spsSeriesRLCBranchLib/Series RLC Branch  LConnTagsString=__new0  RConnTagsString=__new0  BranchType=L  Resistance=Shunt.R  Inductance=Shunt.L  SetiL0=off  InitialCurrent=0  Capacitance=1e-6  Setx0=off  InitialVoltage=0  Measurements=None
  Series RLC Branch3 : spsSeriesRLCBranchLib/Series RLC Branch  LConnTagsString=__new0  RConnTagsString=__new0  BranchType=R  Resistance=Shunt.R  Inductance=Shunt.L  SetiL0=off  InitialCurrent=0  Capacitance=1e-6  Setx0=off  InitialVoltage=0  Measurements=None
  Voltage Measurement{1,3..5} (4 alike) : spsVoltageMeasurementLib/Voltage Measurement  PhasorSimulation=off  OutputType=Complex  PSBequivalent=0
  - : PMIOPort  Side=Left
  1 : PMIOPort  Port=2  Side=Left
  2 : PMIOPort  Port=3  Side=Left
  3 : PMIOPort  Port=4  Side=Left
  Iabc_lowside_shunt : Outport
  Iabc_lowside : Outport  Port=2
  Iabc_lowside_shunt1_sample : Outport  Port=3
  Iabc_lowside_sample : Outport  Port=4
  Div : Outport  Port=5
  tag scope: i_shunt_sample=global
  wires:
  Gain2/1 -> Mux1/3
  Voltage Measurement3/1 -> Gain/1
  Current Measurement/1 -> Mux/1
  Current Measurement2/1 -> Mux/3
  Gain1/1 -> Mux1/2
  Gain/1 -> Mux1/1
  Mux1/1 -> Sample time2/1(In1), Iabc_lowside_shunt/1
  Current Measurement1/1 -> Mux/2
  Voltage Measurement4/1 -> Gain1/1
  Voltage Measurement5/1 -> Scope/2, Gain2/1
  Mux/1 -> Sample time2/2(In2), Iabc_lowside/1
  Sample time2/1(Out1) -> [i_shunt_sample], Iabc_lowside_shunt1_sample/1
  Sample time2/2(Out2) -> Iabc_lowside_sample/1
  Sample time2/3(Div) -> Gain3/1  "Div"
  Gain3/1 -> Div/1  "div'"
  Voltage Measurement1/1 -> Scope/1
  Current Measurement3/1 -> Scope/3
  [S2] -> Scope/4
  connections:
  Current Measurement2/RConn1 -- Voltage Measurement5/LConn1 -- Series RLC Branch2/LConn1
  Current Measurement2/LConn1 -- Ground/LConn1 -- Current Measurement1/LConn1 -- Current Measurement/LConn1 -- -/RConn1
  Current Measurement1/RConn1 -- Voltage Measurement4/LConn1 -- Series RLC Branch1/LConn1
  Series RLC Branch1/RConn1 -- Voltage Measurement4/LConn2 -- 2/RConn1
  Series RLC Branch/RConn1 -- Voltage Measurement3/LConn2 -- 1/RConn1
  Current Measurement/RConn1 -- Voltage Measurement3/LConn1 -- Series RLC Branch/LConn1
  Voltage Measurement5/LConn2 -- Current Measurement3/RConn1 -- Series RLC Branch3/RConn1 -- Voltage Measurement1/LConn2
  Voltage Measurement1/LConn1 -- Series RLC Branch3/LConn1 -- Series RLC Branch2/RConn1
  Current Measurement3/LConn1 -- 3/RConn1

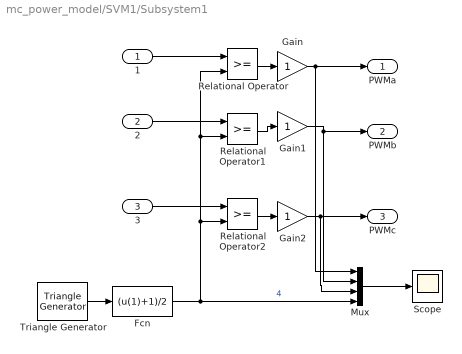
== system mc_power_model/SVM1/Subsystem1 ==
  1 : Inport
  2 : Inport  Port=2
  3 : Inport  Port=3
  Fcn : Fcn  Expr=(u(1)+1)/2
  Gain : Gain  OutDataTypeStr=double
  Gain1 : Gain  OutDataTypeStr=double
  Gain2 : Gain  OutDataTypeStr=double
  Mux : Mux
  Relational Operator : RelationalOperator  OutDataTypeStr=boolean  RndMeth=Simplest  InputSameDT=off
  Relational Operator1 : RelationalOperator  OutDataTypeStr=boolean  RndMeth=Simplest  InputSameDT=off
  Relational Operator2 : RelationalOperator  OutDataTypeStr=boolean  RndMeth=Simplest  InputSameDT=off
  Scope : Scope
  Triangle Generator : spsTriangleGeneratorLib/Triangle Generator  Freq=f_s  Phase=180  Ts=0
  PWMa : Outport  VectorParamsAs1DForOutWhenUnconnected=off
  PWMb : Outport  Port=2  VectorParamsAs1DForOutWhenUnconnected=off
  PWMc : Outport  Port=3  VectorParamsAs1DForOutWhenUnconnected=off
  wires:
  Relational Operator/1 -> Gain/1
  2/1 -> Relational Operator1/1
  Relational Operator1/1 -> Gain1/1
  Triangle Generator/1 -> Fcn/1
  Relational Operator2/1 -> Gain2/1
  3/1 -> Relational Operator2/1
  1/1 -> Relational Operator/1
  Fcn/1 -> Mux/4, Relational Operator2/2, Relational Operator1/2, Relational Operator/2  "4"
  Mux/1 -> Scope/1
  Gain/1 -> Mux/1, PWMa/1
  Gain1/1 -> Mux/2, PWMb/1
  Gain2/1 -> Mux/3, PWMc/1

== system mc_power_model/SVM1/abc to ab ==
  Us : Inport  PortDimensions=3
  alpha : Fcn  Expr=(2*u[1]-u[2]-u[3])/3
  beta : Fcn  Expr=(u[2]-u[3])/sqrt(3)
  U_alpha : Outport  VectorParamsAs1DForOutWhenUnconnected=off
  U_beta : Outport  Port=2  VectorParamsAs1DForOutWhenUnconnected=off
  wires:
  beta/1 -> U_beta/1
  Us/1 -> alpha/1, beta/1
  alpha/1 -> U_alpha/1

== system mc_power_model/SVM1/alpha_beta2abc ==
  alpha : Inport
  beta : Inport  Port=2
  Mux : Mux  Inputs=2
  a-cal : Fcn  Expr=u(1)
  b-cal : Fcn  Expr=(-u(1) + sqrt(3)*u(2))/2
  c-cal : Fcn  Expr=(-u(1) - sqrt(3)*u(2))/2
  a : Outport  VectorParamsAs1DForOutWhenUnconnected=off
  b : Outport  Port=2  VectorParamsAs1DForOutWhenUnconnected=off
  c : Outport  Port=3  VectorParamsAs1DForOutWhenUnconnected=off
  wires:
  alpha/1 -> Mux/1
  beta/1 -> Mux/2
  Mux/1 -> b-cal/1, c-cal/1, a-cal/1
  a-cal/1 -> a/1
  b-cal/1 -> b/1
  c-cal/1 -> c/1

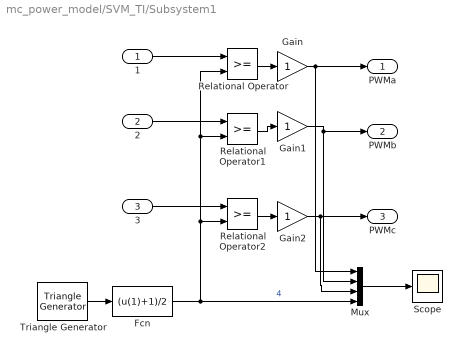
== system mc_power_model/SVM_TI/Subsystem1 ==
  1 : Inport
  2 : Inport  Port=2
  3 : Inport  Port=3
  Fcn : Fcn  Expr=(u(1)+1)/2
  Gain : Gain  OutDataTypeStr=double
  Gain1 : Gain  OutDataTypeStr=double
  Gain2 : Gain  OutDataTypeStr=double
  Mux : Mux
  Relational Operator : RelationalOperator  OutDataTypeStr=boolean  RndMeth=Simplest  InputSameDT=off
  Relational Operator1 : RelationalOperator  OutDataTypeStr=boolean  RndMeth=Simplest  InputSameDT=off
  Relational Operator2 : RelationalOperator  OutDataTypeStr=boolean  RndMeth=Simplest  InputSameDT=off
  Scope : Scope
  Triangle Generator : spsTriangleGeneratorLib/Triangle Generator  Freq=f_s  Phase=180  Ts=0
  PWMa : Outport  VectorParamsAs1DForOutWhenUnconnected=off
  PWMb : Outport  Port=2  VectorParamsAs1DForOutWhenUnconnected=off
  PWMc : Outport  Port=3  VectorParamsAs1DForOutWhenUnconnected=off
  wires:
  Relational Operator/1 -> Gain/1
  2/1 -> Relational Operator1/1
  Relational Operator1/1 -> Gain1/1
  Triangle Generator/1 -> Fcn/1
  Relational Operator2/1 -> Gain2/1
  3/1 -> Relational Operator2/1
  1/1 -> Relational Operator/1
  Fcn/1 -> Mux/4, Relational Operator2/2, Relational Operator1/2, Relational Operator/2  "4"
  Mux/1 -> Scope/1
  Gain/1 -> Mux/1, PWMa/1
  Gain1/1 -> Mux/2, PWMb/1
  Gain2/1 -> Mux/3, PWMc/1

== system mc_power_model/Stator current controller/Decoupling ==
  pi_d_out : Inport
  id : Inport  Port=2
  we : Inport  Port=3
  iq : Inport  Port=4
  pi_q_out : Inport  Port=5
  Decoupling : Subsystem
  Sum2 : Sum  Inputs=|++
  Sum3 : Sum  Inputs=++|
  vdff : Outport  VectorParamsAs1DForOutWhenUnconnected=off
  vqff : Outport  Port=2  VectorParamsAs1DForOutWhenUnconnected=off
  wires:
  pi_d_out/1 -> Sum2/1
  Sum2/1 -> vdff/1
  Sum3/1 -> vqff/1
  pi_q_out/1 -> Sum3/2
  Decoupling/2(VqFF) -> Sum3/1
  we/1 -> Decoupling/3(we)
  Decoupling/1(VdFF) -> Sum2/2
  id/1 -> Decoupling/1(Id)
  iq/1 -> Decoupling/2(Iq)

== system mc_power_model/Stator current controller/Rid ==
  error : Inport
  input_saturation : Inport  Port=2
  out_saturation : Inport  Port=3
  Add : Sum
  Integrator : Integrator
  Subtract : Sum  Inputs=|+-
  Subtract2 : Sum  Inputs=|+-
  k_i : Gain  Gain=Ki_id
  k_p : Gain  Gain=Kp_id
  kc : Gain  Gain=1/Kp_id
  Out1 : Outport  VectorParamsAs1DForOutWhenUnconnected=off
  wires:
  Subtract2/1 -> k_i/1
  k_i/1 -> Integrator/1
  k_p/1 -> Add/1
  Integrator/1 -> Add/2
  error/1 -> Subtract2/1, k_p/1
  kc/1 -> Subtract2/2
  Subtract/1 -> kc/1
  Add/1 -> Out1/1
  out_saturation/1 -> Subtract/2
  input_saturation/1 -> Subtract/1

== system mc_power_model/Stator current controller/Riq ==
  Error : Inport
  input_saturation : Inport  Port=2
  out_saturation : Inport  Port=3
  Add1 : Sum
  Gain : Gain  Gain=Kp_iq
  Gain1 : Gain  Gain=Ki_iq
  Integrator1 : Integrator
  Subtract1 : Sum  Inputs=|+-
  Subtract3 : Sum  Inputs=|+-
  kc1 : Gain  Gain=1/Kp_iq
  Out1 : Outport  VectorParamsAs1DForOutWhenUnconnected=off
  wires:
  Subtract1/1 -> kc1/1
  Gain1/1 -> Integrator1/1
  Integrator1/1 -> Add1/2
  Gain/1 -> Add1/1
  Subtract3/1 -> Gain1/1
  Error/1 -> Gain/1, Subtract3/1
  kc1/1 -> Subtract3/2
  input_saturation/1 -> Subtract1/1
  out_saturation/1 -> Subtract1/2
  Add1/1 -> Out1/1

== system mc_power_model/Stator current controller/Saturation ==
  Vd_ref : Inport
  Vs_max : Inport  Port=2
  Vq_ref : Inport  Port=3
  Saturation Dynamic1 : simulink/Discontinuities/Saturation Dynamic  OutMin=[]  OutMax=[]  OutDataTypeStr=Inherit: Same as second input  OutDataType=fixdt(1, 16)  OutScaling=2^-10  DoSatur=off
  Saturation Dynamic2 : simulink/Discontinuities/Saturation Dynamic  OutMin=[]  OutMax=[]  OutDataTypeStr=Inherit: Same as second input  OutDataType=fixdt(1, 16)  OutScaling=2^-10  DoSatur=off
  chia deu : Subsystem
  uu tien truc d : Subsystem
  uu tien truc d1_modify1 : Subsystem
  uu tien truc d1_modify2 : Subsystem
  uu tien truc q : Subsystem
  Vd_sat : Outport  VectorParamsAs1DForOutWhenUnconnected=off
  Vq_sat : Outport  Port=2  VectorParamsAs1DForOutWhenUnconnected=off
  wires:
  Vd_ref/1 -> uu tien truc d1_modify1/2(vd_ref), Saturation Dynamic1/2
  Vq_ref/1 -> uu tien truc d1_modify1/3(vq_ref), Saturation Dynamic2/2
  Saturation Dynamic2/1 -> Vq_sat/1
  Vs_max/1 -> uu tien truc d1_modify1/1(vs_max)
  uu tien truc d1_modify1/2(vd_low) -> Saturation Dynamic1/3
  Saturation Dynamic1/1 -> Vd_sat/1
  uu tien truc d1_modify1/4(vq_low) -> Saturation Dynamic2/3
  uu tien truc d1_modify1/1(vd_up) -> Saturation Dynamic1/1
  uu tien truc d1_modify1/3(vq_up) -> Saturation Dynamic2/1

== system mc_power_model/CONVERTER/Subsystem/Sample time ==
  4 : Inport
  Pulse Generator : DiscretePulseGenerator  PulseType=Time based  Period=1/f_s  PulseWidth=50
  Subsystem : Subsystem
  Iabc_lowside_shunt1 : Outport
  wires:
  Subsystem/1(Out1) -> Iabc_lowside_shunt1/1
  Pulse Generator/1 -> Subsystem/Trigger
  4/1 -> Subsystem/1(4)

== system mc_power_model/CONVERTER/Subsystem/Sample time1 ==
  4 : Inport
  Pulse Generator : DiscretePulseGenerator  PulseType=Time based  Period=1/f_s  PulseWidth=50
  Subsystem : Subsystem
  Iabc_lowside_cm1 : Outport
  wires:
  Subsystem/1(Out1) -> Iabc_lowside_cm1/1
  Pulse Generator/1 -> Subsystem/Trigger
  4/1 -> Subsystem/1(4)

== system mc_power_model/CONVERTER/Subsystem/Sample time2 ==
  In1 : Inport
  In2 : Inport  Port=2
  Pulse Generator : DiscretePulseGenerator  PulseType=Time based  Period=1/f_s  PulseWidth=50
  Subsystem : Subsystem
  Out1 : Outport
  Out2 : Outport  Port=2
  Div : Outport  Port=3
  wires:
  Subsystem/1(Out1) -> Out1/1
  Pulse Generator/1 -> Subsystem/Trigger
  In1/1 -> Subsystem/1(4)
  In2/1 -> Subsystem/2(1)
  Subsystem/2(Iabc_lowside_shunt2) -> Out2/1
  Subsystem/3(Iabc_lowside_shunt3) -> Div/1

== system mc_power_model/Stator current controller/Decoupling/Decoupling ==
  note: VqFF = Ld*Id*we + Phi*we
  note: VdFF = -Lq*Iq*we
  Id : Inport
  Iq : Inport  Port=2
  we : Inport  Port=3
  Constant : Constant  Value=Lq
  Constant1 : Constant  Value=Ld
  Constant2 : Constant  Value=Phi
  Gain1 : Gain  Gain=-1
  Product{,1..3} (4 alike) : Product
  Sum : Sum  Inputs=|++
  VdFF : Outport  VectorParamsAs1DForOutWhenUnconnected=off
  VqFF : Outport  Port=2  VectorParamsAs1DForOutWhenUnconnected=off
  wires:
  Product2/1 -> VqFF/1
  Gain1/1 -> VdFF/1
  Product/1 -> Product3/1
  Product3/1 -> Gain1/1
  Constant/1 -> Product/2
  Iq/1 -> Product/1
  Id/1 -> Product1/1
  Constant1/1 -> Product1/2
  Sum/1 -> Product2/1
  Constant2/1 -> Sum/2
  Product1/1 -> Sum/1
  we/1 -> Product2/2, Product3/2

== system mc_power_model/Stator current controller/Saturation/chia deu ==
  vs_max : Inport
  vd_ref : Inport  Port=2
  vq_ref : Inport  Port=3
  limit vd : MATLAB Function  TreatAsAtomicUnit=on
  limit vq : MATLAB Function  TreatAsAtomicUnit=on
  vd_up : Outport  VectorParamsAs1DForOutWhenUnconnected=off
  vd_low : Outport  Port=2  VectorParamsAs1DForOutWhenUnconnected=off
  vq_up : Outport  Port=3  VectorParamsAs1DForOutWhenUnconnected=off
  vq_low : Outport  Port=4  VectorParamsAs1DForOutWhenUnconnected=off
  wires:
  vq_ref/1 -> limit vd/3(vq_ref), limit vq/3(vq_ref)
  vd_ref/1 -> limit vd/2(vd_ref), limit vq/2(vd_ref)
  vs_max/1 -> limit vd/1(v_max), limit vq/1(v_max)
  limit vq/1(vq_up) -> vq_up/1
  limit vq/2(vq_low) -> vq_low/1
  limit vd/1(vd_up) -> vd_up/1
  limit vd/2(vd_low) -> vd_low/1

== system mc_power_model/Stator current controller/Saturation/uu tien truc d ==
  vs_max : Inport
  vd_ref : Inport  Port=2
  vq_ref : Inport  Port=3
  limit vq : MATLAB Function  TreatAsAtomicUnit=on
  vd_up : Outport  VectorParamsAs1DForOutWhenUnconnected=off
  vd_low : Outport  Port=2  VectorParamsAs1DForOutWhenUnconnected=off
  vq_up : Outport  Port=3  VectorParamsAs1DForOutWhenUnconnected=off
  vq_low : Outport  Port=4  VectorParamsAs1DForOutWhenUnconnected=off
  wires:
  limit vq/2(vq_low) -> vq_low/1
  limit vq/1(vq_up) -> vq_up/1
  vs_max/1 -> limit vq/1(v_max)
  vd_ref/1 -> limit vq/2(vd_ref)
  vq_ref/1 -> limit vq/3(vq_ref)
  limit vq/3(vd_up) -> vd_up/1
  limit vq/4(vd_low) -> vd_low/1

== system mc_power_model/Stator current controller/Saturation/uu tien truc d1_modify1 ==
  vs_max : Inport
  vd_ref : Inport  Port=2
  vq_ref : Inport  Port=3
  limit vq : MATLAB Function  TreatAsAtomicUnit=on
  vd_up : Outport  VectorParamsAs1DForOutWhenUnconnected=off
  vd_low : Outport  Port=2  VectorParamsAs1DForOutWhenUnconnected=off
  vq_up : Outport  Port=3  VectorParamsAs1DForOutWhenUnconnected=off
  vq_low : Outport  Port=4  VectorParamsAs1DForOutWhenUnconnected=off
  wires:
  limit vq/2(vq_low) -> vq_low/1
  limit vq/1(vq_up) -> vq_up/1
  vs_max/1 -> limit vq/1(v_max)
  vd_ref/1 -> limit vq/2(vd_ref)
  vq_ref/1 -> limit vq/3(vq_ref)
  limit vq/3(vd_up) -> vd_up/1
  limit vq/4(vd_low) -> vd_low/1

== system mc_power_model/Stator current controller/Saturation/uu tien truc d1_modify2 ==
  vs_max : Inport
  vd_ref : Inport  Port=2
  vq_ref : Inport  Port=3
  limit vq : MATLAB Function  TreatAsAtomicUnit=on
  vd_up : Outport  VectorParamsAs1DForOutWhenUnconnected=off
  vd_low : Outport  Port=2  VectorParamsAs1DForOutWhenUnconnected=off
  vq_up : Outport  Port=3  VectorParamsAs1DForOutWhenUnconnected=off
  vq_low : Outport  Port=4  VectorParamsAs1DForOutWhenUnconnected=off
  wires:
  limit vq/4(vd_low) -> vd_low/1
  limit vq/3(vd_up) -> vd_up/1
  vq_ref/1 -> limit vq/3(vq_ref)
  vd_ref/1 -> limit vq/2(vd_ref)
  vs_max/1 -> limit vq/1(v_max)
  limit vq/1(vq_up) -> vq_up/1
  limit vq/2(vq_low) -> vq_low/1

== system mc_power_model/Stator current controller/Saturation/uu tien truc q ==
  vs_max : Inport
  vd_ref : Inport  Port=2
  vq_ref : Inport  Port=3
  limit vq : MATLAB Function  TreatAsAtomicUnit=on
  vd_up : Outport  VectorParamsAs1DForOutWhenUnconnected=off
  vd_low : Outport  Port=2  VectorParamsAs1DForOutWhenUnconnected=off
  vq_up : Outport  Port=3  VectorParamsAs1DForOutWhenUnconnected=off
  vq_low : Outport  Port=4  VectorParamsAs1DForOutWhenUnconnected=off
  wires:
  limit vq/2(vq_low) -> vq_low/1
  limit vq/1(vq_up) -> vq_up/1
  vs_max/1 -> limit vq/1(v_max)
  vd_ref/1 -> limit vq/2(vd_ref)
  vq_ref/1 -> limit vq/3(vq_ref)
  limit vq/3(vd_up) -> vd_up/1
  limit vq/4(vd_low) -> vd_low/1

== system mc_power_model/CONVERTER/Subsystem/Sample time/Subsystem ==
  4 : Inport
  Trigger : TriggerPort  VariantControl=(inherit)  PortDimensions=1
  Out1 : Outport
  wires:
  4/1 -> Out1/1

== system mc_power_model/CONVERTER/Subsystem/Sample time1/Subsystem ==
  4 : Inport
  Trigger : TriggerPort  VariantControl=(inherit)  PortDimensions=1
  Out1 : Outport
  wires:
  4/1 -> Out1/1

== system mc_power_model/CONVERTER/Subsystem/Sample time2/Subsystem ==
  4 : Inport
  1 : Inport  Port=2
  Trigger : TriggerPort  VariantControl=(inherit)  PortDimensions=1
  Divide : Product  Inputs=*/
  Out1 : Outport
  Iabc_lowside_shunt2 : Outport  Port=2
  Iabc_lowside_shunt3 : Outport  Port=3
  wires:
  4/1 -> Divide/1, Out1/1
  1/1 -> Divide/2, Iabc_lowside_shunt2/1
  Divide/1 -> Iabc_lowside_shunt3/1

== matlab function mc_power_model/Battery current estimator (S)/Estimate ibattery ==
  data: id_fb input; ibat_etm output; iq_fb input; ud_sp input; uq_sp input; udc input
function ibat_etm = fcn(id_fb, iq_fb, ud_sp , uq_sp, udc)
us_sp = sqrt(ud_sp*ud_sp + uq_sp*uq_sp);
is_fb = sqrt(id_fb*id_fb + iq_fb*iq_fb);
if ((id_fb+iq_fb) < 0)
    is_fb = -is_fb;
end
ibat_etm = is_fb * us_sp / udc * 1.5;
end

== matlab function mc_power_model/Stator current controller/Saturation/chia deu/limit vd ==
  data: v_max input; vd_ref input; vq_ref input; vd_up output; vd_low output
function [vd_up,vd_low] = fcn(v_max,vd_ref, vq_ref)
vd = v_max*vd_ref/sqrt(vd_ref*vd_ref+vq_ref*vq_ref); 
if( vd > 0 )
    vd_up = vd;
    vd_low = 0;
else 
    vd_up = 0;
    vd_low = vd;
end

== matlab function mc_power_model/Stator current controller/Saturation/chia deu/limit vq ==
  data: v_max input; vd_ref input; vq_ref input; vq_up output; vq_low output
function [vq_up,vq_low] = fcn(v_max,vd_ref, vq_ref)
vq = v_max*vq_ref/sqrt(vd_ref*vd_ref+vq_ref*vq_ref); 
if( vq > 0 )
    vq_up = vq;
    vq_low = 0;
else 
    vq_up = 0;
    vq_low = vq;
end

== matlab function mc_power_model/Stator current controller/Saturation/uu tien truc d/limit vq ==
  data: v_max input; vd_ref input; vq_ref input; vq_up output; vq_low output; vd_up output; vd_low output
function [vq_up, vq_low , vd_up, vd_low] = fcn(v_max,vd_ref, vq_ref) 
%saturation d axis
if( vd_ref > 0 )
    vd_up = v_max;
    vd_low = 0;
else 
    vd_up = 0;
    vd_low = -v_max;
end
%saturation q axis
if( vd_ref > v_max )
    vd = v_max;
elseif (vd_ref < - v_max)
    vd = -v_max;
else
    vd = vd_ref;  
end

vq_max = sqrt(v_max*v_max - vd*vd);
if( vq_ref > 0 )
    vq_up = vq_max;
    vq_low = 0;
else 
    vq_up = 0;
    vq_low = -vq_max;
end

end

== matlab function mc_power_model/Stator current controller/Saturation/uu tien truc d1_modify1/limit vq ==
  data: v_max input; vd_ref input; vq_ref input; vq_up output; vq_low output; vd_up output; vd_low output
function [vq_up, vq_low , vd_up, vd_low] = fcn(v_max,vd_ref, vq_ref) 
%saturation d axis
    vd_up = v_max;
    vd_low = -v_max;
%saturation q axis
if( vd_ref > v_max )
    vd = v_max;
elseif (vd_ref < - v_max)
    vd = -v_max;
else
    vd = vd_ref;  
end

vq_max = sqrt(v_max*v_max - vd*vd);
vq_up = vq_max;
vq_low = -vq_max;
end

== matlab function mc_power_model/MATLAB Function ==
  data: vd input; vs output; vq input
function vs = fcn(vd, vq)

vs = sqrt(vd^2+vq^2);

== matlab function mc_power_model/Stator current controller/Saturation/uu tien truc d1_modify2/limit vq ==
  data: v_max input; vd_ref input; vq_ref input; vq_up output; vq_low output; vd_up output; vd_low output
function [vq_up, vq_low , vd_up, vd_low] = fcn(v_max,vd_ref, vq_ref) 
%saturation d axis
    vd_up = v_max;
    vd_low = -v_max;
%saturation q axis
if( vd_ref > v_max )
    vd = v_max;
elseif (vd_ref < - v_max)
    vd = -v_max;
else
    vd = vd_ref;  
end

vq_max = sqrt(v_max*v_max - vd*vd);
vq_up = vq_max;
vq_low = -vq_max;
end

== matlab function mc_power_model/SVM_TI/fcn ==
  data: v_alpha input; v_beta input; vdc input; duty_a output; duty_b output; duty_c output; limit_duty input
function [duty_a, duty_b, duty_c] = fcn(v_alpha, v_beta, vdc, limit_duty)

va_tmp = 0.5*(-v_alpha/vdc);
vb_tmp = sqrt(3)/2*(v_beta/vdc);

va = v_alpha;
vb = va_tmp + vb_tmp;
vc = va_tmp - vb_tmp;

v_max = 0;
v_min = 0;

if va > vb
    v_max = va;
    v_min = vb;
else
    v_max = vb;
    v_min = va;
end

if vc> v_max
    v_max = vc;
elseif vc < v_min
    v_min = vc;
end

v_com = (v_max + v_min)/2;

duty_a = va - v_com +0.5*limit_duty;
duty_b = va - v_com +0.5*limit_duty;
duty_c = va - v_com +0.5*limit_duty;

== matlab function mc_power_model/Stator current controller/Saturation/uu tien truc q/limit vq ==
  data: v_max input; vd_ref input; vq_ref input; vq_up output; vq_low output; vd_up output; vd_low output
function [vq_up, vq_low , vd_up, vd_low] = fcn(v_max,vd_ref, vq_ref) 
%saturation d axis
if( vq_ref > 0 )
    vq_up = v_max;
    vq_low = 0;
else 
    vq_up = 0;
    vq_low = -v_max;
end
%saturation q axis
if( vq_ref > v_max )
    vq = v_max;
elseif (vq_ref < - v_max)
    vq = -v_max;
else
    vq = vq_ref;  
end

vd_max = sqrt(v_max*v_max - vq*vq);
if( vd_ref > 0 )
    vd_up = vd_max;
    vd_low = 0;
else 
    vd_up = 0;
    vd_low = -vd_max;
end

end

== matlab function mc_power_model/Battery current estimator(P)/Estimate ibattery ==
  data: id_fb input; ibat_etm output; iq_fb input; ud_sp input; uq_sp input; udc input
function ibat_etm = fcn(id_fb, iq_fb, ud_sp , uq_sp, udc)

ibat_etm = 1.5*(id_fb * ud_sp + iq_fb * uq_sp )/udc;
end

== matlab function mc_power_model/MATLAB Function1 ==
  data: id input; is output; iq input
function is = fcn(id, iq)

is = sqrt(id^2+iq^2);

== matlab function mc_power_model/SVM_TI/MATLAB Function3 ==
  data: du input; i_q_limit output; dv input; dw input; i_bat_limit input
function i_q_limit = fcn(du,dv,dw,i_bat_limit)
dmax = du;
dmin = du;
if dv > dmax
    dmax = dv;
end
if dw > dmax
    dmax = dw;
end
if dv < dmin
    dmin = dv;
end
if dw < dmin
    dmin = dw;
end
i_q_limit = i_bat_limit/(dmax-dmin);
end

== matlab function mc_power_model/MATLAB Function2 ==
  data: vs input; i output; is input; ia input
function i = fcn(vs, is, ia)

i = (((-8*10^-5*ia+0.2057)*vs/is)+1)*ia ;

== matlab function mc_power_model/SVM1/He so dieu che IGBT da db dc ==
  data: sec input; d1 input; d2 input; d0 input; da output; db output; dc output
function [da, db, dc]=d_abc(sec, d1, d2, d0)
da = inf; db = inf; dc = inf;

if sec == 1
    da = 1 - d0/2; db = 1 - (d0/2 + d1); dc = 1 - (d0/2 + d1 + d2);
elseif sec == 2
    da = 1 - (d0/2 + d1); db = 1 - d0/2; dc = 1 - (d0/2 + d1 + d2);
elseif sec == 3
    da = 1- (d0/2 + d1 + d2); db = 1 - d0/2; dc = 1 - (d0/2 + d1);
elseif sec == 4
    da = 1 - (d0/2 + d1 + d2); db = 1 - (d0/2 + d1); dc = 1 - d0/2;
elseif sec == 5
    da = 1 - (d0/2 + d1); db = 1 - (d0/2 + d1 + d2); dc = 1 - d0/2;
elseif sec == 6
    da = 1 - d0/2; db = 1 - (d0/2 + d1 + d2); dc = 1 - (d0/2 + d1);
end

== matlab function mc_power_model/SVM1/He so dieu che Vecto Us d1 d2 d0 ==
  data: Sec input; u_alpha input; u_beta input; Vdc input; d1 output; d2 output; d0 output
function [d1, d2, d0] = d1d2d0(Sec, u_alpha, u_beta, Vdc)


A1 = (1/Vdc)*[3/2, -(sqrt(3))/2; 0, sqrt(3)];
A2 = (1/Vdc)*[-3/2, (sqrt(3))/2; 3/2, (sqrt(3))/2];
A3 = (1/Vdc)*[0, sqrt(3); -3/2, -(sqrt(3))/2];
A4 = (1/Vdc)*[0, -sqrt(3); -3/2, (sqrt(3))/2];
A5 = (1/Vdc)*[-3/2, -(sqrt(3))/2; 3/2, -(sqrt(3))/2];
A6 = (1/Vdc)*[3/2, (sqrt(3))/2; 0, -sqrt(3)];

if Sec == 1
    d12 = A1*[u_alpha; u_beta];
elseif Sec ==2
    d12 = A2*[u_alpha; u_beta];
elseif Sec == 3
    d12 = A3*[u_alpha; u_beta];
elseif Sec == 4
    d12 = A4*[u_alpha; u_beta];
elseif Sec == 5
    d12 = A5*[u_alpha; u_beta];
else
    d12 = A6*[u_alpha; u_beta];
end
d1 = d12(1); d2 = d12(2);
d0 = 1 - d1 - d2;

== matlab function mc_power_model/SVM1/MATLAB Function3 ==
  data: du input; i_q_limit output; dv input; dw input; i_bat_limit input
function i_q_limit = fcn(du,dv,dw,i_bat_limit)
dmax = du;
dmin = du;
if dv > dmax
    dmax = dv;
end
if dw > dmax
    dmax = dw;
end
if dv < dmin
    dmin = dv;
end
if dw < dmin
    dmin = dw;
end
i_q_limit = i_bat_limit/(dmax-dmin);
end

== matlab function mc_power_model/SVM1/Xac dinh Sector ==
  data: Us input; sec output
function sec = Sector(Us)
%i-clarke
u_a = Us(1);
u_b = Us(2);
u_c = Us(3);

if u_a >= u_b
    if u_b >= u_c
        sec = 1;
    else
        if u_c >= u_a
            sec = 5;
        else sec = 6;
        end
    end
else
    if u_b < u_c
        sec = 4;
    else
        if u_c < u_a
            sec = 2;
        else sec = 3;
        end
    end
end
